simulink model "Assignment_model_2"  (R2017a)
settings: Solver=ode45  StartTime=0.0  StopTime=100  RelTol=1e-3  EnableMultiTasking=on
settings Model: Creator=Administrator  LastModifiedBy=sarthakbhagat
settings DataIOCC: LimitDataPoints=on  SaveFormat=Array
settings OptimizationCC: LifeSpan=inf
settings DebuggingCC: SolverPrmCheckMsg=warning  AllowSymbolicDim=off  SFUnexpectedBacktrackingDiag=warning  SFNoUnconditionalDefaultTransitionDiag=warning  SFExecutionAtInitializationDiag=none
settings HardwareCC: ProdBitPerPointer=32  ProdBitPerSizeT=32  ProdBitPerPtrDiffT=32  ProdLargestAtomicFloat=None  ProdIntDivRoundTo=Undefined  ProdEndianess=Unspecified  ProdWordSize=32  ProdHWDeviceType=32-bit Generic
settings ModelReferenceCC: PropagateSignalLabelsOutOfModel=off
settings GRTTargetCC: TargetLangStandard=C89/C90 (ANSI)  GeneratePreprocessorConditionals=Disable all
settings ConfigComp: CovMetricSettings=dw  CovHtmlReporting=on  CovSaveCumulativeToWorkspaceVar=on  CovSaveSingleToWorkspaceVar=on  CovExternalEMLEnable=off  CovSFcnEnable=off

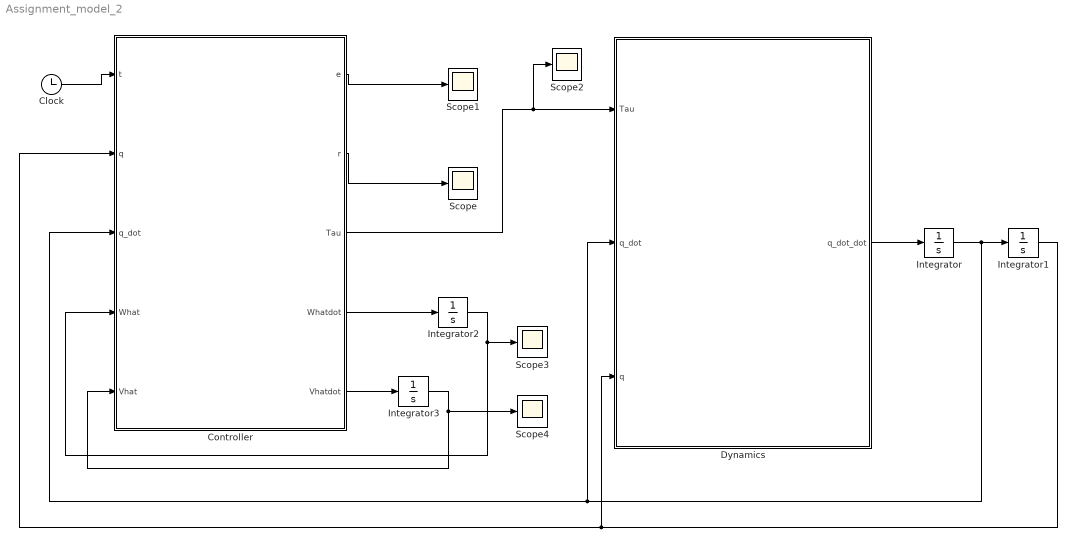
== system Assignment_model_2 ==
  Clock : Clock
      settings: Decimation=50
  Controller : MATLAB Function  TreatAsAtomicUnit=on
  Dynamics : MATLAB Function  TreatAsAtomicUnit=on
  Integrator : Integrator  InitialCondition=[1;-1]
  Integrator1 : Integrator  InitialCondition=[1,1]
  Integrator2 : Integrator  InitialCondition=rand(21,2)
  Integrator3 : Integrator  InitialCondition=rand(7,20)
  Scope{,1..4} (5 alike) : Scope
  wires:
  Dynamics/1(q_dot_dot) -> Integrator/1
  Integrator/1 -> Dynamics/2(q_dot), Controller/3(q_dot), Integrator1/1
  Integrator1/1 -> Controller/2(q), Dynamics/3(q)
  Controller/3(Tau) -> Scope2/1, Dynamics/1(Tau)
  Clock/1 -> Controller/1(t)
  Controller/4(Whatdot) -> Integrator2/1
  Integrator2/1 -> Controller/4(What), Scope3/1
  Controller/1(e) -> Scope1/1
  Controller/2(r) -> Scope/1
  Controller/5(Vhatdot) -> Integrator3/1
  Integrator3/1 -> Scope4/1, Controller/5(Vhat)

== matlab function Assignment_model_2/Controller ==
  data: e output; r output; Tau output; t input; q input; q_dot input; What input; Whatdot output; Vhat input; Vhatdot output
function [e,r,Tau, Whatdot, Vhatdot] = controller(t,q,q_dot, What, Vhat)

alpha=1;
k=1;

qd=[0.5*sin(t);2*cos(t/4)];
qd_dot=[0.5*cos(t);-0.5*sin(t/4)];
qd_ddot=[-0.5*sin(t);-0.25*cos(t/4)];
e=q-qd;     %Tracking Error
e_dot=q_dot-qd_dot;

r=e_dot+alpha*e;         %Filtered Tracking Error

%----------------------------------------------------------%

X=[qd' qd_dot' qd_ddot']';
L=20; % number of neurons
phi=zeros(L,1);
Vr=5*eye(size(X,1)); % variance of RBF

persistent C; % centroids of RBF

if isempty (C)
    C=-1+2*rand(size(X,1),L);
end


for i=1:L
    phi(i,1)=exp(-((X-C(:,i))'*(Vr\(X-C(:,i)))));
end
phi_bar=[1;phi];
k1 = 5;

%%%% Normal
%Whatdot=eye(L+1)*phi_bar*r';

%%%% Sigma mod
%Whatdot=eye(L+1)*phi_bar*r' - k1*eye(L+1)*What;

%%%% e mod
%norm_z = norm([e]);
%Whatdot=eye(L+1)*phi_bar*r' - k1*norm_z*eye(L+1)*What;

%%%% Multilayer NN
%%%% NOTE: taken gamma_v and gamma_w as identity

X_d_bar = [1;X];

sigmoid1 = 1 ./ ( 1 + exp(-Vhat'*X_d_bar));
sigmoid_1_bar = [1;sigmoid1];
sigmoid_derivative = diag(sigmoid1)*(eye(L) - diag(sigmoid1));
sigmoid_derivative_bar = [ones(1,L);sigmoid_derivative];

k_w = 1;
Whatdot = (sigmoid_1_bar - sigmoid_derivative_bar*Vhat'*X_d_bar)*r' - k_w*What;

k_v = 1;
Vhatdot = X_d_bar*r'*What'*sigmoid_derivative_bar - k_v*Vhat;

Tau=-What'*sigmoid_1_bar-k*r-e;   % Controller

== matlab function Assignment_model_2/Dynamics ==
  data: Tau input; q_dot_dot output; q_dot input; q input
function q_dot_dot   = dynamics(Tau,q_dot,q)
%#codegen
p1=3.473;
p2=0.196;
p3=0.242;
fd1=5.3;
fd2=1.1;

c2=cos(q(2));
s2=sin(q(2));
% alpha=1;

M=[p1+2*p3*c2 p2+p3*c2;p2+p3*c2 p2];% Inertia matrix
Vm=[-p3*s2*q_dot(2) -p3*s2*(q_dot(1)+q_dot(2));p3*s2*q_dot(1) 0];%Centripetal coriolis matrix
fd=[fd1 0;0 fd2]; % Friction matrix
q_dot_dot=-M\(Vm*q_dot+fd*q_dot-Tau);   %EL dynamics
